simulink model "GearSelect_Testrig"  (R2019a)
settings: Solver=VariableStepDiscrete  StartTime=0.0  StopTime=inf  RelTol=1e-3  EnableMultiTasking=on
PostLoadFcn:
  | set_param([bdroot '/Signals/p'],'Value','0');
  | set_param([bdroot '/Signals/m'],'Value','0');
  | set_param([bdroot '/Signals/g'],'Value','0');
  | %warning('off', 'sl3d:interface:enginewarn')
  | %open_system([bdroot '/Anim']);
  | GearSelectorGUI
libraries: Animation_Lib x1
Description:
  | Copyright 2014-2019 The MathWorks, Inc.
settings Model: Creator=smiller  LastModifiedBy=smiller
settings DataIOCC: LimitDataPoints=on  SaveFormat=Array  SignalLoggingSaveFormat=ModelDataLogs  ReturnWorkspaceOutputs=off
settings OptimizationCC: ExpressionDepthLimit=2147483647  LifeSpan=inf
settings DebuggingCC: UnderspecifiedInitializationDetection=Classic  MergeDetectMultiDrivingBlocksExec=none  SolverPrmCheckMsg=warning  FcnCallInpInsideContextMsg=warning  AllowSymbolicDim=off  StateNameClashWarn=warning  PregeneratedLibrarySubsystemCodeDiagnostic=none  SFUnexpectedBacktrackingDiag=warning  SFNoUnconditionalDefaultTransitionDiag=warning  SFExecutionAtInitializationDiag=none  ArithmeticOperatorsInVariantConditions=warning
settings HardwareCC: ProdBitPerPointer=32  ProdBitPerSizeT=32  ProdBitPerPtrDiffT=32  ProdLargestAtomicFloat=None  ProdIntDivRoundTo=Undefined  ProdEndianess=Unspecified  ProdWordSize=32  ProdHWDeviceType=32-bit Generic
settings ModelReferenceCC: PropagateSignalLabelsOutOfModel=off
settings SFSimCC: SimUseLocalCustomCode=off
settings RTWCC: RTWUseLocalCustomCode=off
settings CodeAppCC: StateflowObjectComments=on
settings GRTTargetCC: TargetLangStandard=C89/C90 (ANSI)  GeneratePreprocessorConditionals=Disable all  CombineOutputUpdateFcns=off  GRTInterface=on
settings ConfigComp: CovMetricSettings=dw  CovHtmlReporting=on  CovSaveCumulativeToWorkspaceVar=on  CovSaveSingleToWorkspaceVar=on  CovExternalEMLEnable=off  CovSFcnEnable=off

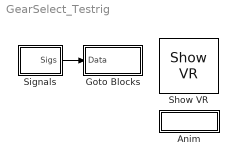
== system GearSelect_Testrig ==
  Anim : Subsystem
      settings: OpenFcn=|
      | vrblk = find_system(bdroot,'LookUnderMasks','all','FollowLinks','on','Name','VR Sink');
      | if(~isempty(vrblk))
      | open_system(vrblk);
      | close_system(get_param(vrblk,'Parent'));
      | end
      mask Display: disp('Anim')
  Goto Blocks : Subsystem
  Show VR : Animation_Lib/Show VR  SystemSampleTime=-1
  Signals : Subsystem
  wires:
  Signals/1(Sigs) -> Goto Blocks/1(Data)

== system GearSelect_Testrig/Anim ==

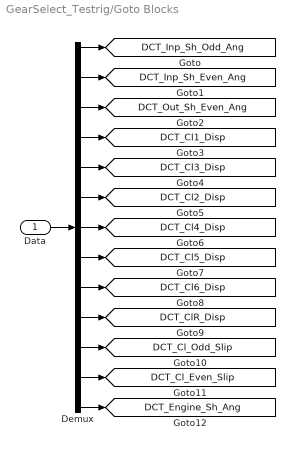
== system GearSelect_Testrig/Goto Blocks ==
  Data : Inport
  Demux : Demux  Outputs=13
  tag scope: DCT_Cl1_Disp=global, DCT_Cl2_Disp=global, DCT_Cl3_Disp=global, DCT_Cl4_Disp=global, DCT_Cl5_Disp=global, DCT_Cl6_Disp=global, DCT_ClR_Disp=global, DCT_Cl_Even_Slip=global, DCT_Cl_Odd_Slip=global, DCT_Engine_Sh_Ang=global, DCT_Inp_Sh_Even_Ang=global, DCT_Inp_Sh_Odd_Ang=global, DCT_Out_Sh_Even_Ang=global
  wires:
  Data/1 -> Demux/1
  Demux/4 -> [DCT_Cl1_Disp]
  Demux/5 -> [DCT_Cl3_Disp]
  Demux/6 -> [DCT_Cl2_Disp]
  Demux/7 -> [DCT_Cl4_Disp]
  Demux/8 -> [DCT_Cl5_Disp]
  Demux/9 -> [DCT_Cl6_Disp]
  Demux/10 -> [DCT_ClR_Disp]
  Demux/11 -> [DCT_Cl_Odd_Slip]
  Demux/12 -> [DCT_Cl_Even_Slip]
  Demux/13 -> [DCT_Engine_Sh_Ang]
  Demux/3 -> [DCT_Out_Sh_Even_Ang]
  Demux/2 -> [DCT_Inp_Sh_Even_Ang]
  Demux/1 -> [DCT_Inp_Sh_Odd_Ang]

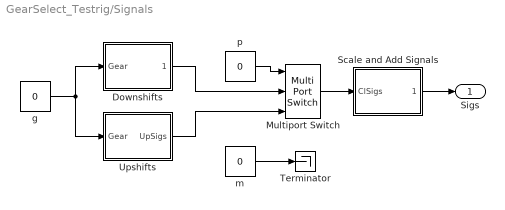
== system GearSelect_Testrig/Signals ==
  Downshifts : Subsystem
  Multiport Switch : MultiPortSwitch  DataPortOrder=Zero-based contiguous  Inputs=2  zeroidx=on
  Scale and Add Signals : Subsystem
  Terminator : Terminator
  Upshifts : Subsystem
  g : Constant  Value=0
  m : Constant  Value=0
  p : Constant  Value=0
  Sigs : Outport
  wires:
  p/1 -> Multiport Switch/1
  g/1 -> Upshifts/1(Gear), Downshifts/1(Gear)
  m/1 -> Terminator/1
  Downshifts/1(DwnSigs) -> Multiport Switch/2
  Upshifts/1(UpSigs) -> Multiport Switch/3
  Multiport Switch/1 -> Scale and Add Signals/1(ClSigs)
  Scale and Add Signals/1(AllSigs) -> Sigs/1

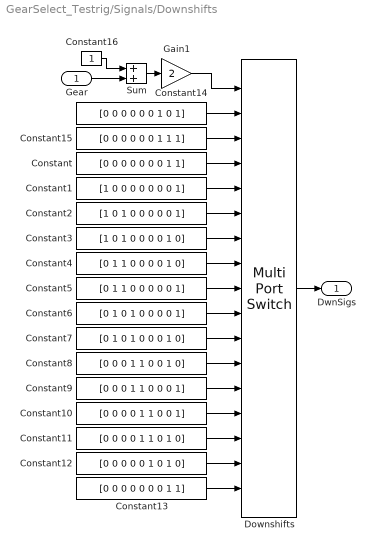
== system GearSelect_Testrig/Signals/Downshifts ==
  Gear : Inport
  Constant : Constant  Value=[0 0 0 0 0 0 0 1 1]
  Constant1 : Constant  Value=[1 0 0 0 0 0 0 0 1]
  Constant10 : Constant  Value=[0 0 0 0 1 1 0 0 1]
  Constant11 : Constant  Value=[0 0 0 0 1 1 0 1 0]
  Constant12 : Constant  Value=[0 0 0 0 0 1 0 1 0]
  Constant13 : Constant  Value=[0 0 0 0 0 0 0 1 1]
  Constant14 : Constant  Value=[0 0 0 0 0 0 1 0 1]
  Constant15 : Constant  Value=[0 0 0 0 0 0 1 1 1]
  Constant16 : Constant
  Constant2 : Constant  Value=[1 0 1 0 0 0 0 0 1]
  Constant3 : Constant  Value=[1 0 1 0 0 0 0 1 0]
  Constant4 : Constant  Value=[0 1 1 0 0 0 0 1 0]
  Constant5 : Constant  Value=[0 1 1 0 0 0 0 0 1]
  Constant6 : Constant  Value=[0 1 0 1 0 0 0 0 1]
  Constant7 : Constant  Value=[0 1 0 1 0 0 0 1 0]
  Constant8 : Constant  Value=[0 0 0 1 1 0 0 1 0]
  Constant9 : Constant  Value=[0 0 0 1 1 0 0 0 1]
  Downshifts : MultiPortSwitch  DataPortOrder=Zero-based contiguous  Inputs=15  DataPortForDefault=Additional data port  zeroidx=on
  Gain1 : Gain  Gain=2
  Sum : Sum
  DwnSigs : Outport
  wires:
  Downshifts/1 -> DwnSigs/1
  Gear/1 -> Sum/2
  Constant13/1 -> Downshifts/17
  Constant12/1 -> Downshifts/16
  Constant11/1 -> Downshifts/15
  Constant10/1 -> Downshifts/14
  Constant9/1 -> Downshifts/13
  Constant8/1 -> Downshifts/12
  Constant7/1 -> Downshifts/11
  Constant6/1 -> Downshifts/10
  Constant5/1 -> Downshifts/9
  Constant4/1 -> Downshifts/8
  Constant3/1 -> Downshifts/7
  Constant2/1 -> Downshifts/6
  Constant1/1 -> Downshifts/5
  Constant/1 -> Downshifts/4
  Constant14/1 -> Downshifts/2
  Constant15/1 -> Downshifts/3
  Constant16/1 -> Sum/1
  Sum/1 -> Gain1/1
  Gain1/1 -> Downshifts/1

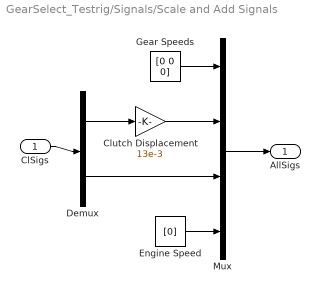
== system GearSelect_Testrig/Signals/Scale and Add Signals ==
  ClSigs : Inport
  Clutch Displacement : Gain  Gain=13e-3
  Demux : Demux  Outputs=[7 2]
  Engine Speed : Constant  Value=[0]
  Gear Speeds : Constant  Value=[0 0 0]
  Mux : Mux
  AllSigs : Outport
  wires:
  Mux/1 -> AllSigs/1
  ClSigs/1 -> Demux/1
  Demux/1 -> Clutch Displacement/1
  Clutch Displacement/1 -> Mux/2
  Gear Speeds/1 -> Mux/1
  Demux/2 -> Mux/3
  Engine Speed/1 -> Mux/4

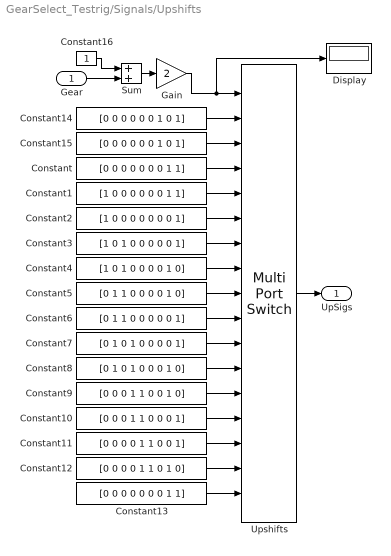
== system GearSelect_Testrig/Signals/Upshifts ==
  Gear : Inport
  Constant : Constant  Value=[0 0 0 0 0 0 0 1 1]
  Constant1 : Constant  Value=[1 0 0 0 0 0 0 1 1]
  Constant10 : Constant  Value=[0 0 0 1 1 0 0 0 1]
  Constant11 : Constant  Value=[0 0 0 0 1 1 0 0 1]
  Constant12 : Constant  Value=[0 0 0 0 1 1 0 1 0]
  Constant13 : Constant  Value=[0 0 0 0 0 0 0 1 1]
  Constant14 : Constant  Value=[0 0 0 0 0 0 1 0 1]
  Constant15 : Constant  Value=[0 0 0 0 0 0 1 0 1]
  Constant16 : Constant
  Constant2 : Constant  Value=[1 0 0 0 0 0 0 0 1]
  Constant3 : Constant  Value=[1 0 1 0 0 0 0 0 1]
  Constant4 : Constant  Value=[1 0 1 0 0 0 0 1 0]
  Constant5 : Constant  Value=[0 1 1 0 0 0 0 1 0]
  Constant6 : Constant  Value=[0 1 1 0 0 0 0 0 1]
  Constant7 : Constant  Value=[0 1 0 1 0 0 0 0 1]
  Constant8 : Constant  Value=[0 1 0 1 0 0 0 1 0]
  Constant9 : Constant  Value=[0 0 0 1 1 0 0 1 0]
  Display : Display
  Gain : Gain  Gain=2
  Sum : Sum
  Upshifts : MultiPortSwitch  DataPortOrder=Zero-based contiguous  Inputs=15  DataPortForDefault=Additional data port  zeroidx=on
  UpSigs : Outport
  wires:
  Constant/1 -> Upshifts/4
  Constant1/1 -> Upshifts/5
  Constant2/1 -> Upshifts/6
  Constant3/1 -> Upshifts/7
  Constant4/1 -> Upshifts/8
  Constant5/1 -> Upshifts/9
  Constant6/1 -> Upshifts/10
  Constant7/1 -> Upshifts/11
  Constant8/1 -> Upshifts/12
  Constant9/1 -> Upshifts/13
  Constant10/1 -> Upshifts/14
  Constant11/1 -> Upshifts/15
  Constant12/1 -> Upshifts/16
  Constant13/1 -> Upshifts/17
  Upshifts/1 -> UpSigs/1
  Gain/1 -> Display/1, Upshifts/1
  Constant14/1 -> Upshifts/2
  Constant15/1 -> Upshifts/3
  Constant16/1 -> Sum/1
  Gear/1 -> Sum/2
  Sum/1 -> Gain/1
